simulink model "TPTLFAD"  (R2019b)
settings: Solver=VariableStepAuto  StartTime=0.0  StopTime=10.0  RelTol=1e-3
undefined symbols (not defined in the file): sigbuilder_block
libraries: powerlib x21, powerlib_meascontrol x1
settings Model: Creator=mdeat  LastModifiedBy=mdeat

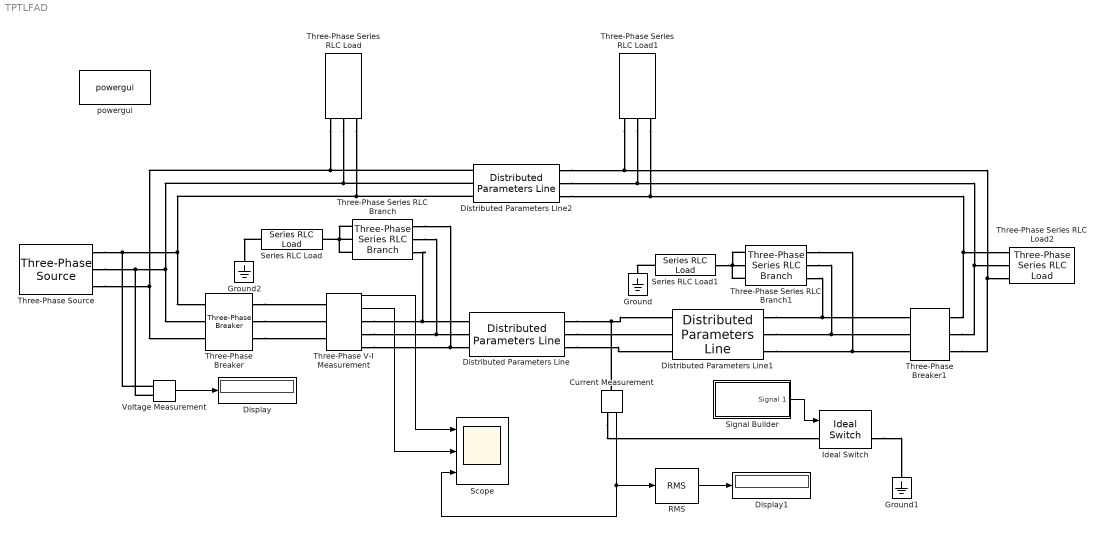
== system TPTLFAD ==
  Current Measurement : powerlib/Measurements/Current Measurement  PhasorSimulation=off  OutputType=Complex  PSBequivalent=0
      settings: SourceProductName=Simscape Electrical
  Display : Display
  Display1 : Display
      settings: Decimation=3
  Distributed Parameters Line : powerlib/Elements/Distributed Parameters Line  Phases=3  Frequency=50  Resistance=[0.01273 0.3864]  Inductance="[0.9337e-3  4.1264e-3]"  Capacitance=[12.74e-9 7.751e-9]  Length=100  x1=[-0.0006 -0.38452520954395 6685.93509775308 -17741.9769006427;-0.00055 -0.387585149283488 6963.78458325206 -17634.7656233459;-0.0005 -0.390549458187001 7239.91585910648 -17523.2032315063;-0.00045 -0.393417404855623 7514.26079405584 -17407.3172514746;-0.0004 -0.396188281666429 7786.75169759257 -17287.1362763824;-0.00035 -0.398861404947025 8057.32133666358 -17162.6899590869;-0.0003 -0.401436115144242 8325.90295225906 -17034.0090048549;-0.00025 -0.403911776986865 8592.43027588424 -16901.1251637863;-0.0002 -0.406287779642378 8856.83754591013 -16764.0712229804;-0.00015 -0.408563536867679 9119.05952379927 -16622.8809984465;-0.0001 -0.410738487153726 9379.03151020233 -16477.5893267598;-5e-05 -0.412812093864078 9636.68936092171 -16328.2320564661]  x2=[-0.0006 -5.92316789265769 5456.31459715794 -14466.7927612595;-0.00055 -5.97612134191109 5682.85304062556 -14379.2789098277;-0.0005 -6.027600272646 5907.98932513977 -14288.2171864867;-0.00045 -6.07759198320656 6131.66790169114 -14193.6300593541;-0.0004 -6.12608413888622 6353.83358093789 -14095.5408663883;-0.00035 -6.17306477497117 6574.43154682299 -13993.9738096297;-0.0003 -6.21852229969245 6793.40737009924 -13888.95394923;-0.00025 -6.26244549708603 7010.70702175886 -13780.5071972681;-0.0002 -6.30482352976019 7226.27688636432 -13668.6603113575;-0.00015 -6.34564594156947 7440.06377527717 -13553.4408880436;-0.0001 -6.38490266019462 7652.01493978154 -13434.8773559951;-5e-05 -6.42258399962771 7862.07808409907 -13312.9989689894]  x3=[-0.0006 0.0104881362628189 130.695383780921 -20.0395154301661;-0.00055 0.00977436823662447 130.993279666128 -17.9847488637507;-0.0005 0.00905818853132463 131.258854919672 -15.9255448296648;-0.00045 0.00833977385354527 131.492044014833 -13.8624114056911;-0.0004 0.00761930146135826 131.692789415691 -11.7958576391308;-0.00035 0.00689694912054572 131.861041591322 -9.72639342120331;-0.0003 0.00617289506073895 131.99675902802 -7.65452936123825;-0.00025 0.00544731793144295 132.099908239537 -5.58077666069048;-0.0002 0.00472039675795733 132.17046377535 -3.50564698700865;-0.00015 0.00399231089720451 132.208408226935 -1.42965234738889;-0.0001 0.00326323999347602 132.213732232067 0.64669503755524;-5e-05 0.00253336393410806 132.186434477127 2.72288286017556]  x4=[-0.0006 -0.0183664652402812 -92.4379896808149 -100.943098545329;-0.00055 -0.0177383067669422 -90.8404000022742 -102.381915870777;-0.0005 -0.0171057716318325 -89.220396814307 -103.795471990458;-0.00045 -0.0164690159035318 -87.5783798284593 -105.183418130549;-0.0004 -0.0158281966919881 -85.9147541878524 -106.545411836111;-0.00035 -0.015183472109753 -84.2299303672197 -107.881117055575;-0.0003 -0.01453500123297 -82.5243240716283 -109.190204223665;-0.00025 -0.0138829440621247 -80.7983561339103 -110.472350342711;-0.0002 -0.013227461482567 -79.052452410828 -111.727239062344;-0.00015 -0.0125687152248152 -77.2870436780006 -112.954560757548;-0.0001 -0.0119068678246514 -75.5025655236164 -114.154012605061;-5e-05 -0.0112420825830182 -73.6994582409585 -115.325298658087]  x5=0.000565541566995743  V1=[0.5493 1.86e+04 1.86e+04;314.2 314.2 314.2;-2.813 0.7306 -0.8402]  V2=[6.715 1.266e+04 1.266e+04;314.2 314.2 314.2;-2.012 0.732 -0.8387]  I1=[0.04661 207.4 207.3;314.2 314.2 314.2;3.055 2.006 0.4351]  I2=[0.0429 211.8 211.7;314.2 314.2 314.2;-0.2798 -0.579 -2.15]  nHarmo=1  Measurements=None
      settings: SourceProductName=Simscape Electrical
  Distributed Parameters Line1 : powerlib/Elements/Distributed Parameters Line  Phases=3  Frequency=50  Resistance=[0.01273 0.3864]  Inductance="[0.9337e-3  4.1264e-3]"  Capacitance=[12.74e-9 7.751e-9]  Length=100  x1=[-0.0006 -5.92316789265769 5456.31459715794 -14466.7927612595;-0.00055 -5.97612134191109 5682.85304062556 -14379.2789098277;-0.0005 -6.027600272646 5907.98932513977 -14288.2171864867;-0.00045 -6.07759198320656 6131.66790169114 -14193.6300593541;-0.0004 -6.12608413888622 6353.83358093789 -14095.5408663883;-0.00035 -6.17306477497117 6574.43154682299 -13993.9738096297;-0.0003 -6.21852229969245 6793.40737009924 -13888.95394923;-0.00025 -6.26244549708603 7010.70702175886 -13780.5071972681;-0.0002 -6.30482352976019 7226.27688636432 -13668.6603113575;-0.00015 -6.34564594156947 7440.06377527717 -13553.4408880436;-0.0001 -6.38490266019462 7652.01493978154 -13434.8773559951;-5e-05 -6.42258399962771 7862.07808409907 -13312.9989689894]  x2=[-0.0006 -2.4818772730336 4172.61390055077 -11017.6777013695;-0.00055 -2.51614242875928 4345.14790500093 -10950.7678161331;-0.0005 -2.54978676399051 4516.60980922338 -10881.1559927979;-0.00045 -2.582801977491 4686.95730755889 -10808.8594070397;-0.0004 -2.61517992325084 4856.1483693112 -10733.8958969592;-0.00035 -2.6469126124964 5024.1412491175 -10656.2839586809;-0.0003 -2.67799221566143 5190.89449724841 -10576.0427417892;-0.00025 -2.7084110643189 5356.36696983515 -10493.1920446037;-0.0002 -2.73816165307307 5520.51783902112 -10407.7523092942;-0.00015 -2.76723664141135 5683.3066030356 -10319.7446168369;-0.0001 -2.7956288555154 5844.69309618691 -10229.190681813;-5e-05 -2.82333129003125 6004.63749877277 -10136.1128470511]  x3=[-0.0006 -0.00877207086275021 132.591416429137 -5.5658318383681;-0.00055 -0.00843835895449951 132.662922732132 -3.48196363483196;-0.0005 -0.00810256500744266 132.701696444021 -1.39723630887066;-0.00045 -0.00776477187371151 132.70772799797 0.687835764242553;-0.0004 -0.00742506289870729 132.681015905785 2.77273812417325;-0.00035 -0.00708352190053642 132.621566758273 4.85695635246118;-0.0003 -0.00674023314932961 132.529395223622 6.93997619944534;-0.00025 -0.00639528134644947 132.404524043781 9.02128371114738;-0.0002 -0.00604875160359174 132.246984028842 11.1003653560821;-0.00015 -0.00570072942178524 132.056814049449 13.1767081519634;-0.0001 -0.00535130067029576 131.834061027198 15.2497997922757;-5e-05 -0.00500055156543912 131.578779923063 17.3191287726768]  x4=[-0.0006 -0.0016306409798328 -102.241302778118 -90.1634387758921;-0.00055 -0.0020950101745643 -100.813029255366 -91.758655324782;-0.0005 -0.00255886245688353 -99.3598816261422 -93.3312317984847;-0.00045 -0.00302208337818061 -97.8822184328813 -94.8807801872862;-0.0004 -0.00348455864562453 -96.3804042668652 -96.4069181633082;-0.00035 -0.00394617415036321 -94.8548096782672 -97.9092691748411;-0.0003 -0.00440681599567816 -93.3058110847241 -99.3874625392529;-0.00025 -0.00486637052508678 -91.7337906784606 -100.84113353445;-0.0002 -0.00532472435038539 -90.1391363319894 -102.269923488865;-0.00015 -0.00578176437962612 -88.5222415024091 -103.673479869957;-0.0001 -0.00623737784502056 -86.8835051343249 -105.051456371191;-5e-05 -0.00669145233076364 -85.2233315614145 -106.403512997484]  x5=0.000565541566995743  V1=[6.715 1.266e+04 1.266e+04;314.2 314.2 314.2;-2.012 0.732 -0.8387]  V2=[5.474 6566 6567;314.2 314.2 314.2;-2.358 0.7374 -0.8333]  I1=[0.009569 208.3 208.3;314.2 314.2 314.2;0.4179 2.115 0.5446]  I2=[0.02481 210.8 210.8;314.2 314.2 314.2;-2.432 -0.6867 -2.257]  nHarmo=1  Measurements=None
      settings: SourceProductName=Simscape Electrical
  Distributed Parameters Line2 : powerlib/Elements/Distributed Parameters Line  Phases=3  Frequency=50  Resistance=[0.01273 0.3864]  Inductance="[0.9337e-3  4.1264e-3]"  Capacitance=[12.74e-9 7.751e-9]  Length=100  x1=[-0.0006 -0.384537693929809 18707.8773158488 3081.51212528889;-0.00055 -0.387596917092123 18753.9655845588 2787.28314490684;-0.0005 -0.390560506514882 18795.4265928825 2492.36644411581;-0.00045 -0.39342773097674 18832.2501109363 2196.83478919876;-0.0004 -0.396197883032965 18864.4270530683 1900.76109816943;-0.00035 -0.398870279189988 18891.9494800994 1604.21842278082;-0.0003 -0.401444260074045 18914.8106012826 1307.27993050083;-0.00025 -0.403919190593868 18933.0047759784 1010.01888645923;-0.0002 -0.406294460097385 18946.5275150463 712.508635370638;-0.00015 -0.408569482522387 18955.3754819528 414.822583437764;-0.0001 -0.410743696541133 18959.5464935945 117.034180239549;-5e-05 -0.412816565698847 18959.0395208368 -180.783099391419]  x2=[-0.0006 -2.48196803456183 11627.5697352464 1897.69772174902;-0.00055 -2.51623014916185 11655.9295765043 1714.82876419717;-0.0005 -2.54987142162372 11681.4134915505 1531.53669830728;-0.00045 -2.58288355146685 11704.0151926105 1347.86674865396;-0.0004 -2.61525839344217 11723.7291030527 1163.86423304897;-0.00035 -2.64698795954186 11740.5503587646 979.574551359751;-0.0003 -2.67806442097026 11754.4748093531 795.043174307674;-0.00025 -2.70848011007553 11765.4990191683 610.315632248822;-0.0002 -2.7382275222415 11773.6202681516 425.437503940062;-0.00015 -2.76729931773933 11778.8365525061 240.454405293163;-0.0001 -2.79568832353849 11781.1465851918 55.4119781197545;-5e-05 -2.82338753507661 11780.5497962427 -129.644121130108]  x3=[-0.0006 0.00911023101475099 98.1013585417015 -227.49394331378;-0.00055 0.00881103040446518 94.515949219262 -229.006527205494;-0.0005 0.00850965580426935 90.9072195006253 -230.462607163318;-0.00045 0.00820618157383654 87.2760597858507 -231.861823921311;-0.0004 0.0079006825908921 83.6233660092636 -233.203832243674;-0.00035 0.00759323423273882 79.950039418397 -234.488301009935;-0.0003 0.00728391235765861 76.2569863516221 -235.714913296646;-0.00025 0.00697279328619567 72.5451180145227 -236.883366455578;-0.0002 0.0066599537823255 68.8153502550691 -237.9933721884;-0.00015 0.00634547103451458 65.0686033376462 -239.044656617805;-0.0001 0.00602942263667521 61.3058017159922 -240.036960355092;-5e-05 0.00571188656902042 57.5278738051032 -240.970038564161]  x4=[-0.0006 -0.0126006940175466 12.5640693369541 251.883998673451;-0.00055 -0.0123560390485514 16.5188576294362 251.655338301593;-0.0005 -0.0121083354118084 20.4695701409752 251.36458574061;-0.00045 -0.0118576442244834 24.4152320923747 251.011812729343;-0.0004 -0.0116040273408758 28.3548699505884 250.597106309256;-0.00035 -0.0113475473371566 32.2875116689247 250.120568802953;-0.0003 -0.0110882674959289 36.2121869268852 249.582317788931;-0.00025 -0.010826251790614 40.1279273695761 248.982486072576;-0.0002 -0.0105615648696664 44.0337668466356 248.321221653387;-0.00015 -0.0102942720406233 47.928741650617 247.598687688465;-0.0001 -0.0100244392539906 51.8118907547694 246.815062452255;-5e-05 -0.00975213308697096 55.6822560501559 245.970539292558]  x5=0.000565541566995743  V1=[0.2351 2.046e+04 2.046e+04;314.2 314.2 314.2;-1.863 1.381 2.952]  V2=[0.1244 1.949e+04 1.949e+04;314.2 314.2 314.2;-2.623 1.095 2.666]  I1=[0.0009912 123.8 123.8;314.2 314.2 314.2;0.3363 -2.155 -0.5845]  I2=[0.001382 268.2 268.2;314.2 314.2 314.2;-2.624 1.095 2.666]  nHarmo=1  Measurements=None
      settings: SourceProductName=Simscape Electrical
  Ground : powerlib/Elements/Ground  LConnTagsString=a
      settings: SourceProductName=Simscape Electrical
  Ground1 : powerlib/Elements/Ground  LConnTagsString=a
      settings: SourceProductName=Simscape Electrical
  Ground2 : powerlib/Elements/Ground  LConnTagsString=a
      settings: SourceProductName=Simscape Electrical
  Ideal Switch : powerlib/Power Electronics/Ideal Switch  Ron=0.001  Lon=0  IC=0  Rs=1e5  Cs=inf  Measurements=on
      settings: SourceProductName=Simscape Electrical
  RMS : powerlib_meascontrol/Measurements/RMS  TrueRMS=on  Freq=50  RMSInit=120  Ts=0
      settings: SourceProductName=Simscape Electrical
  Scope : Scope  NumInputPorts=3
  Series RLC Load : powerlib/Elements/Series RLC Load  LConnTagsString=a  RConnTagsString=__new0  NominalVoltage=1000  NominalFrequency=50  ActivePower=10e3  InductivePower=100  CapacitivePower=100  Setx0=off  InitialVoltage=0  SetiL0=off  InitialCurrent=0  Measurements=None  LoadType=constant Z
      settings: SourceProductName=Simscape Electrical
  Series RLC Load1 : powerlib/Elements/Series RLC Load  LConnTagsString=a  RConnTagsString=__new0  NominalVoltage=1000  NominalFrequency=50  ActivePower=10e3  InductivePower=100  CapacitivePower=100  Setx0=off  InitialVoltage=0  SetiL0=off  InitialCurrent=0  Measurements=None  LoadType=constant Z
      settings: SourceProductName=Simscape Electrical
  Signal Builder : Subsystem  Tag=STV Subsys  LoadFcn=sigbuilder_block('load');  StartFcn=sigbuilder_block('start');  StopFcn=sigbuilder_block('stop');  ClipboardFcn=sigbuilder_block('clipboard');  mask(Sigbuilder block){tuvar=[0:10]}
      mask help: Simulink:masks:SigbuilderBlock_MD
      mask init:
      | if ~strcmp(get_param(bdroot(gcbh),'SimulationStatus'),'stopped') tuvar = sigbuilder_block('maskInit'); end
      settings: CopyFcn=sigbuilder_block('copy');  DeleteFcn=sigbuilder_block('delete');  ModelCloseFcn=sigbuilder_block('modelClose');  PreSaveFcn=sigbuilder_block('preSave');  PauseFcn=sigbuilder_block('pause');  ContinueFcn=sigbuilder_block('continue');  NameChangeFcn=sigbuilder_block('namechange');  OpenFcn=sigbuilder_block('open',[437.6 199.2 550.4 400 ]);  CloseFcn=sigbuilder_block('close');
      mask Display: plot(0, 0, 100, 100,[2, 2, 32, 32, 2], [68, 8, 8, 68, 68],[32, 2], [38, 38], [32, 19, 2],[53, 60, 44], [32, 17, 17, 2],[16, 16, 31, 31]);txt = getActiveGroup(gcbh);text(2, 100, txt,'verticalAlignment', 'top');
  Three-Phase Series RLC Branch : powerlib/Elements/Three-Phase Series RLC Branch  LConnTagsString=A|B|C  RConnTagsString=A|B|C  BranchType=RLC  Resistance=1  Inductance=1e-1  Capacitance=1e-1  Measurements=Branch voltages
      settings: SourceProductName=Simscape Electrical
  Three-Phase Series RLC Branch1 : powerlib/Elements/Three-Phase Series RLC Branch  LConnTagsString=A|B|C  RConnTagsString=A|B|C  BranchType=RLC  Resistance=1  Inductance=1e-1  Capacitance=1e-1  Measurements=Branch voltages
      settings: SourceProductName=Simscape Electrical
  Three-Phase Series RLC Load : powerlib/Elements/Three-Phase Series RLC Load  LConnTagsString=A|B|C  Configuration=Y (grounded)  NominalVoltage=1000  Vabc=[1e3 1e3 1e3]  Vabcp=[1e3 1e3 1e3]  NominalFrequency=50  UnbalancedPower=off  ActivePower=10e1  InductivePower=100  CapacitivePower=100  Pabc=[10e3 9e3 11e3]  QLabc=[100 90 110]  QCabc=[100 90 110]  Pabcp=[10e3 9e3 11e3]  QLabcp=[100 90 110]  QCabcp=[100 90 110]  Measurements=Branch voltages and currents  LoadType=constant Z
      settings: SourceProductName=Simscape Electrical
  Three-Phase Series RLC Load1 : powerlib/Elements/Three-Phase Series RLC Load  LConnTagsString=A|B|C  Configuration=Y (grounded)  NominalVoltage=1000  Vabc=[1e3 1e3 1e3]  Vabcp=[1e3 1e3 1e3]  NominalFrequency=50  UnbalancedPower=off  ActivePower=10e1  InductivePower=100  CapacitivePower=100  Pabc=[10e3 9e3 11e3]  QLabc=[100 90 110]  QCabc=[100 90 110]  Pabcp=[10e3 9e3 11e3]  QLabcp=[100 90 110]  QCabcp=[100 90 110]  Measurements=Branch voltages and currents  LoadType=constant Z
      settings: SourceProductName=Simscape Electrical
  Three-Phase Series RLC Load2 : powerlib/Elements/Three-Phase Series RLC Load  LConnTagsString=A|B|C  Configuration=Y (grounded)  NominalVoltage=1000  Vabc=[1e3 1e3 1e3]  Vabcp=[1e3 1e3 1e3]  NominalFrequency=50  UnbalancedPower=off  ActivePower=10e1  InductivePower=100  CapacitivePower=100  Pabc=[10e3 9e3 11e3]  QLabc=[100 90 110]  QCabc=[100 90 110]  Pabcp=[10e3 9e3 11e3]  QLabcp=[100 90 110]  QCabcp=[100 90 110]  Measurements=Branch voltages and currents  LoadType=constant Z
      settings: SourceProductName=Simscape Electrical
  Three-Phase V-I Measurement : powerlib/Measurements/Three-Phase V-I Measurement  VoltageMeasurement=phase-to-ground  SetLabelV=off  LabelV=Vabc  Vpu=off  VpuLL=off  CurrentMeasurement=yes  SetLabelI=off  LabelI=Iabc  Ipu=off  Pbase=100e6  Vbase=500e3  OutputType=Complex  PhasorSimulation=off  PSBequivalent=0
      settings: SourceProductName=Simscape Electrical
  Three-Phase Breaker : powerlib/Elements/Three-Phase Breaker  InitialState=closed  SwitchA=on  SwitchB=off  SwitchC=on  SwitchTimes="[1/50  5/50]"  External=off  BreakerResistance=0.001  SnubberResistance=1e1  SnubberCapacitance=inf  Measurements=Breaker voltages
      settings: SourceProductName=Simscape Electrical
  Three-Phase Breaker1 : powerlib/Elements/Three-Phase Breaker  InitialState=closed  SwitchA=on  SwitchB=off  SwitchC=on  SwitchTimes="[1/50  5/50]"  External=off  BreakerResistance=0.01  SnubberResistance=1e1  SnubberCapacitance=inf  Measurements=Breaker voltages
      settings: SourceProductName=Simscape Electrical
  Three-Phase Source : powerlib/Electrical Sources/Three-Phase Source  InternalConnection=Yg  VoltagePhases=off  Voltage=25e3  PhaseAngle=0  Voltage_phases=[25e3 25e3 25e3]/sqrt(3)  PhaseAngles_phases=[0 -120 +120]  Frequency=50  NonIdealSource=on  SpecifyImpedance=on  Resistance=0.8929  Inductance=16.58e-3  ShortCircuitLevel=100e6  BaseVoltage=25e3  XRratio=7  BusType=swing  Pref=10e3  Qref=0  Prefabc=[10e3, 10e3, 10e3]  Qrefabc=[0, 0, 0]  Qmin=-inf  Qmax=inf
      settings: SourceProductName=Simscape Electrical
  Voltage Measurement : powerlib/Measurements/Voltage Measurement  PhasorSimulation=off  OutputType=Complex  PSBequivalent=0
      settings: SourceProductName=Simscape Electrical
  powergui : powerlib/powergui  Priority=1  SimulationMode=Discrete  SampleTime=50e-6  frequency=60  Iterations=50  frequencyindice=50  Pbase=100e6  ErrMax=1e-4  UnitsV=kV  UnitsW=MW  buscounter=0  FunctionMessages=off  echomessages=off  EnableUseOfTLC=off  CurrentSourceSwitches=off  DisableSnubberDevices=off  DisableRonSwitches=off  DisableVfSwitches=off  DisplayEquations=off  AutomaticDiscreteSolvers=off  SolverType=Tustin/Backward Euler (TBE)  Interpol=off  ExternalGateDelay=off  methode=off  Ts=100  x0status=blocks  SPID=on  SwTol=0  HookPort=off  NonlinearTolerance=1e-4  nMaxIteration=100  ContinueOnMaxIteration=off  RestoreLinks=warning  ResistiveCurrentMeasurement=off  Frange=[0:2:500]  Ylog=off  Xlog=on  ShowGrid=off  save=off  variable=ZData  structure=0  ZoomFFT=off  StartTime=0.0  cycles=1  DisplayStyle=1  fundamental=60  FreqAxis=off  MaxFrequency=1000  frequencyindicesteady=1  RmsSteady=1  display=off
      settings: SourceProductName=Simscape Electrical
  wires:
  RMS/1 -> Display1/1
  Voltage Measurement/1 -> Display/1
  Three-Phase V-I Measurement/1 -> Scope/1
  Three-Phase V-I Measurement/2 -> Scope/2
  Signal Builder/1(Signal 1) -> Ideal Switch/1
  Current Measurement/1 -> Scope/3, RMS/1
  connections:
  Three-Phase Source/RConn3 -- Three-Phase Series RLC Load/LConn1 -- Distributed Parameters Line2/LConn1 -- Three-Phase Breaker/LConn3
  Three-Phase Source/RConn2 -- Voltage Measurement/LConn2 -- Three-Phase Series RLC Load/LConn2 -- Distributed Parameters Line2/LConn2 -- Three-Phase Breaker/LConn2
  Three-Phase Source/RConn1 -- Voltage Measurement/LConn1 -- Distributed Parameters Line2/LConn3 -- Three-Phase Series RLC Load/LConn3 -- Three-Phase Breaker/LConn1
  Three-Phase Breaker/RConn1 -- Three-Phase V-I Measurement/LConn1
  Three-Phase Breaker/RConn2 -- Three-Phase V-I Measurement/LConn2
  Three-Phase Breaker/RConn3 -- Three-Phase V-I Measurement/LConn3
  Three-Phase V-I Measurement/RConn3 -- Three-Phase Series RLC Branch/RConn1 -- Distributed Parameters Line/LConn3
  Three-Phase V-I Measurement/RConn2 -- Three-Phase Series RLC Branch/RConn2 -- Distributed Parameters Line/LConn2
  Three-Phase V-I Measurement/RConn1 -- Three-Phase Series RLC Branch/RConn3 -- Distributed Parameters Line/LConn1
  Distributed Parameters Line/RConn1 -- Current Measurement/LConn1 -- Distributed Parameters Line1/LConn1
  Distributed Parameters Line/RConn2 -- Distributed Parameters Line1/LConn2
  Distributed Parameters Line/RConn3 -- Distributed Parameters Line1/LConn3
  Distributed Parameters Line1/RConn1 -- Three-Phase Series RLC Branch1/RConn3 -- Three-Phase Breaker1/LConn1
  Distributed Parameters Line1/RConn2 -- Three-Phase Series RLC Branch1/RConn2 -- Three-Phase Breaker1/LConn2
  Distributed Parameters Line1/RConn3 -- Three-Phase Series RLC Branch1/RConn1 -- Three-Phase Breaker1/LConn3
  Current Measurement/RConn1 -- Ideal Switch/LConn1
  Ideal Switch/RConn1 -- Ground1/LConn1
  Series RLC Load1/LConn1 -- Ground/LConn1
  Series RLC Load1/RConn1 -- Three-Phase Series RLC Branch1/LConn3 -- Three-Phase Series RLC Branch1/LConn1 -- Three-Phase Series RLC Branch1/LConn2
  Three-Phase Breaker1/RConn1 -- Three-Phase Series RLC Load1/LConn3 -- Distributed Parameters Line2/RConn3 -- Three-Phase Series RLC Load2/LConn1
  Three-Phase Breaker1/RConn2 -- Three-Phase Series RLC Load1/LConn2 -- Distributed Parameters Line2/RConn2 -- Three-Phase Series RLC Load2/LConn2
  Three-Phase Breaker1/RConn3 -- Distributed Parameters Line2/RConn1 -- Three-Phase Series RLC Load1/LConn1 -- Three-Phase Series RLC Load2/LConn3
  Three-Phase Series RLC Branch/LConn2 -- Series RLC Load/RConn1 -- Three-Phase Series RLC Branch/LConn3 -- Three-Phase Series RLC Branch/LConn1
  Series RLC Load/LConn1 -- Ground2/LConn1

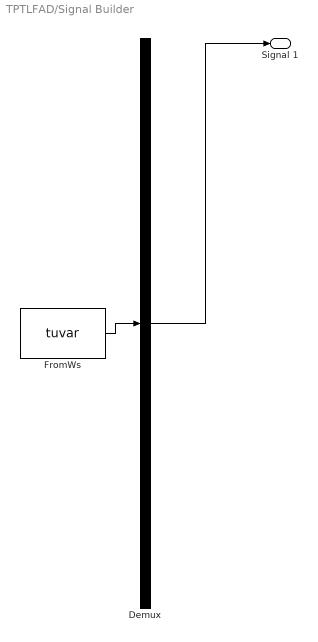
== system TPTLFAD/Signal Builder ==
  Demux : Demux  Tag=STV Demux  Outputs=1
  FromWs : FromWorkspace  Tag=STV FromWs  VariableName=tuvar  SampleTime=0
      SigBuilderData=|
      | common.afterFinalStr = 'Extrapolate'
      | common.sampleTime = 0
      | dataSet.timeRange = [0 10]
      | dataSet.name = 'Group 1'
      | sbobj.Groups.Name = 'Group 1'
      | sbobj.Groups.Signals.Name = 'Signal 1'
      | sbobj.Groups.Signals.XData = [0 4 4 6 6 10]
      | sbobj.Groups.Signals.YData = [0 0 1 1 0 0]
  Signal 1 : Outport  Tag=STV Outport
  wires:
  Demux/1 -> Signal 1/1
  FromWs/1 -> Demux/1
